simulink model "ord2"  (Simulink 10.3)
settings: Solver=ode45  StartTime=0.0  StopTime=40.0  RelTol=1e-3
libraries: simulink x1
settings Model: Creator=iorda  LastModifiedBy=iorda
settings SolverCC: AlgebraicLoopSolver=Auto
settings DataIOCC: SaveFormat=Dataset  SignalLoggingSaveFormat=Dataset  ReturnWorkspaceOutputs=on
settings OptimizationCC: ExpressionDepthLimit=128  LifeSpan=auto
settings DebuggingCC: UnderspecifiedInitializationDetection=Simplified  MergeDetectMultiDrivingBlocksExec=error  FcnCallInpInsideContextMsg=error  StateNameClashWarn=none  SFUnexpectedBacktrackingDiag=error  SFNoUnconditionalDefaultTransitionDiag=error  SFExecutionAtInitializationDiag=warning  SFMachineParentedDataDiag=error  ArithmeticOperatorsInVariantConditions=error
settings HardwareCC: ProdBitPerPointer=64  ProdBitPerSizeT=64  ProdBitPerPtrDiffT=64  ProdLargestAtomicFloat=Float  ProdIntDivRoundTo=Zero  ProdEndianess=LittleEndian  ProdWordSize=64  ProdHWDeviceType=Intel->x86-64 (Windows64)
settings ModelReferenceCC: PropagateSignalLabelsOutOfModel=on
settings SFSimCC: SimUseLocalCustomCode=on  CustomCodeUndefinedFunction=FilterOut
settings RTWCC: RTWUseLocalCustomCode=on
settings CodeAppCC: StateflowObjectComments=off
settings GRTTargetCC: TargetLangStandard=C99 (ISO)  CombineOutputUpdateFcns=on  GRTInterface=off
settings ConfigComp: CovMetricSettings=dwe  CovSaveCumulativeToWorkspaceVar=off  CovSaveSingleToWorkspaceVar=off  CovExternalEMLEnable=on

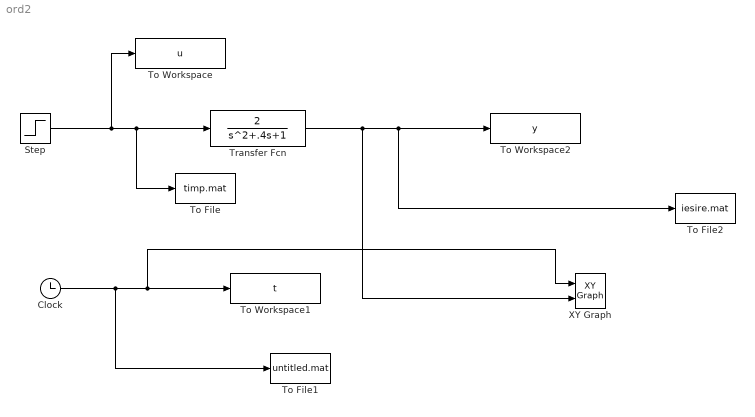
== system ord2 ==
  Clock : Clock
  Step : Step  Time=0  SampleTime=0
  To File : ToFile  Filename=timp.mat  MatrixName=t
  To File1 : ToFile  MatrixName=t
  To File2 : ToFile  Filename=iesire.mat  MatrixName=y
  To Workspace : ToWorkspace  VariableName=u  SampleTime=-1
  To Workspace1 : ToWorkspace  VariableName=t  SaveFormat=Timeseries  SampleTime=-1
      settings: MaxDataPoints=10000
  To Workspace2 : ToWorkspace  VariableName=y  SampleTime=-1
      settings: MaxDataPoints=10000
  Transfer Fcn : TransferFcn  Numerator=[2]  Denominator=[1 .4 1]
  XY Graph : simulink/Sinks/XY Graph  xmin=0  xmax=40  ymin=0  ymax=4  st=-1
  wires:
  Step/1 -> To Workspace/1, To File/1, Transfer Fcn/1
  Transfer Fcn/1 -> XY Graph/2, To File2/1, To Workspace2/1
  Clock/1 -> To File1/1, XY Graph/1, To Workspace1/1
